simulink model "Local_Oscillator"  (R2017a)
settings: Solver=VariableStepAuto  StartTime=0.0  StopTime=0.001  RelTol=1e-3
settings Model: Creator=Alam  LastModifiedBy=Alam

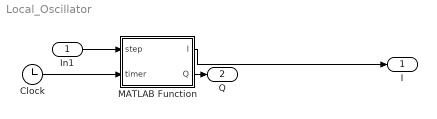
== system Local_Oscillator ==
  In1 : Inport
  Clock : Clock
  MATLAB Function : MATLAB Function  TreatAsAtomicUnit=on
  I : Outport
  Q : Outport  Port=2
  wires:
  In1/1 -> MATLAB Function/1(step)
  Clock/1 -> MATLAB Function/2(timer)
  MATLAB Function/1(I) -> I/1
  MATLAB Function/2(Q) -> Q/1

== matlab function Local_Oscillator/MATLAB Function ==
  data: step input; I output; timer input; Q output
function [I,Q]= Local_Oscillator(step, timer)
f = 9207000+step*500-5000;
I = sin((2*pi*f*timer));
Q = cos((2*pi*f*timer));
